simulink model "Testing_Playground"  (R2022a)
settings: Solver=VariableStepAuto  StartTime=0.0  StopTime=10.0  RelTol=1e-3
libraries: simulink x1
settings Model: Creator=maxju  LastModifiedBy=maxju

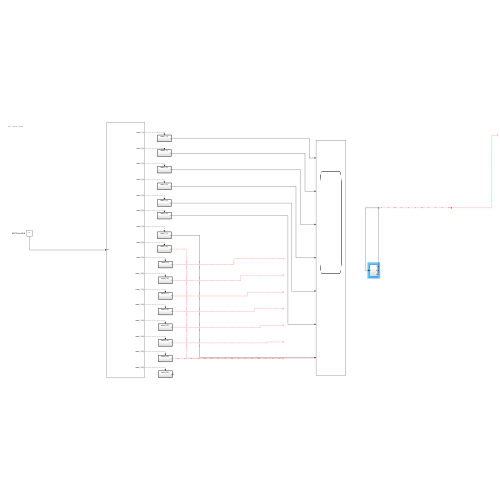
[thumbnail: Simulink's stored preview of the top-level diagram]
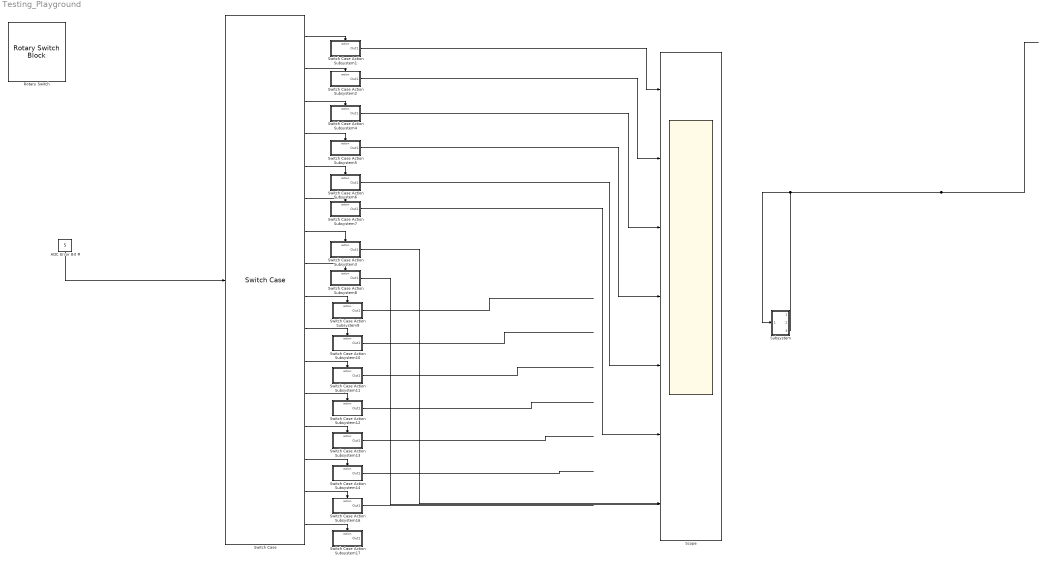
== system Testing_Playground ==
  ADC Error Bit # : Constant  Priority=0  Value=5
  Rotary Switch : RotarySwitchBlock
      settings: Values={{'No Errors', '1', '2', '3', '4', '5', '6', '7', '8', '9', '10', '11', '12', '13', '14', '15', '16'}, [0 1 2 3 4 5 6 7 8 9 10 11 12 13 14 15 16]}
  Scope : Scope  NumInputPorts=7
  Subsystem : Subsystem
  Switch Case : SwitchCase  CaseConditions={1,2,3,4,5,6,7,8,9,10,11,12,13,14,15,16}  ShowDefaultCase=off
  Switch Case Action Subsystem1 : Subsystem  TreatAsAtomicUnit=on
  Switch Case Action Subsystem10 : Subsystem  TreatAsAtomicUnit=on
  Switch Case Action Subsystem11 : Subsystem  TreatAsAtomicUnit=on
  Switch Case Action Subsystem12 : Subsystem  TreatAsAtomicUnit=on
  Switch Case Action Subsystem13 : Subsystem  TreatAsAtomicUnit=on
  Switch Case Action Subsystem14 : Subsystem  TreatAsAtomicUnit=on
  Switch Case Action Subsystem16 : Subsystem  TreatAsAtomicUnit=on
  Switch Case Action Subsystem17 : Subsystem  TreatAsAtomicUnit=on
  Switch Case Action Subsystem2 : Subsystem  TreatAsAtomicUnit=on
  Switch Case Action Subsystem3 : Subsystem  TreatAsAtomicUnit=on
  Switch Case Action Subsystem4 : Subsystem  TreatAsAtomicUnit=on
  Switch Case Action Subsystem5 : Subsystem  TreatAsAtomicUnit=on
  Switch Case Action Subsystem6 : Subsystem  TreatAsAtomicUnit=on
  Switch Case Action Subsystem7 : Subsystem  TreatAsAtomicUnit=on
  Switch Case Action Subsystem8 : Subsystem  TreatAsAtomicUnit=on
  Switch Case Action Subsystem9 : Subsystem  TreatAsAtomicUnit=on
  wires:
  Subsystem/3(Out3) -> Subsystem/1(In1)
  Switch Case Action Subsystem2/1(Out1) -> Scope/2
  Switch Case/10 -> Switch Case Action Subsystem10/Action
  Switch Case/13 -> Switch Case Action Subsystem13/Action
  Switch Case Action Subsystem16/1(Out1) -> ?
  Switch Case Action Subsystem13/1(Out1) -> ?
  Switch Case Action Subsystem9/1(Out1) -> ?
  Switch Case Action Subsystem7/1(Out1) -> Scope/6
  Switch Case/4 -> Switch Case Action Subsystem5/Action
  Switch Case Action Subsystem14/1(Out1) -> ?
  Switch Case/7 -> Switch Case Action Subsystem3/Action
  Switch Case/6 -> Switch Case Action Subsystem7/Action
  Switch Case Action Subsystem6/1(Out1) -> Scope/5
  Switch Case/3 -> Switch Case Action Subsystem4/Action
  Switch Case/15 -> Switch Case Action Subsystem16/Action
  Switch Case/14 -> Switch Case Action Subsystem14/Action
  Switch Case/12 -> Switch Case Action Subsystem12/Action
  Switch Case/5 -> Switch Case Action Subsystem6/Action
  ADC Error Bit #/1 -> Switch Case/1
  Switch Case/9 -> Switch Case Action Subsystem9/Action
  Switch Case/16 -> Switch Case Action Subsystem17/Action
  Switch Case Action Subsystem11/1(Out1) -> ?
  Switch Case Action Subsystem10/1(Out1) -> ?
  Switch Case/11 -> Switch Case Action Subsystem11/Action
  Switch Case Action Subsystem1/1(Out1) -> Scope/1
  Switch Case/2 -> Switch Case Action Subsystem2/Action
  Switch Case Action Subsystem12/1(Out1) -> ?
  Switch Case Action Subsystem4/1(Out1) -> Scope/3
  Switch Case Action Subsystem5/1(Out1) -> Scope/4
  Switch Case/8 -> Switch Case Action Subsystem8/Action
  Switch Case Action Subsystem3/1(Out1) -> Scope/7
  Switch Case Action Subsystem8/1(Out1) -> ?
  Switch Case/1 -> Switch Case Action Subsystem1/Action

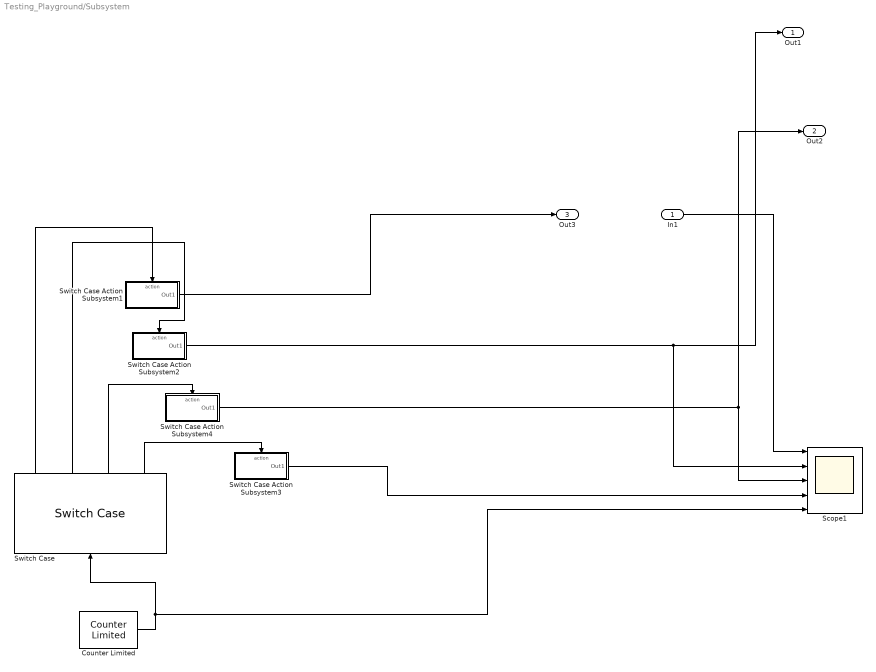
== system Testing_Playground/Subsystem ==
  In1 : Inport
  Counter Limited : simulink/Sources/Counter Limited  uplimit=3  tsamp=1
  Scope1 : Scope  NumInputPorts=5
  Switch Case : SwitchCase  CaseConditions={1,2,3}
  Switch Case Action Subsystem1 : Subsystem  TreatAsAtomicUnit=on
  Switch Case Action Subsystem2 : Subsystem  TreatAsAtomicUnit=on
  Switch Case Action Subsystem3 : Subsystem  TreatAsAtomicUnit=on
  Switch Case Action Subsystem4 : Subsystem  TreatAsAtomicUnit=on
  Out1 : Outport
  Out2 : Outport  Port=2
  Out3 : Outport  Port=3
  wires:
  Switch Case Action Subsystem4/1(Out1) -> Out2/1, Scope1/3
  Switch Case/4 -> Switch Case Action Subsystem3/Action
  Switch Case/2 -> Switch Case Action Subsystem2/Action
  Switch Case/3 -> Switch Case Action Subsystem4/Action
  Switch Case Action Subsystem3/1(Out1) -> Scope1/4
  In1/1 -> Scope1/1
  Switch Case Action Subsystem2/1(Out1) -> Out1/1, Scope1/2
  Switch Case/1 -> Switch Case Action Subsystem1/Action
  Counter Limited/1 -> Scope1/5, Switch Case/1
  Switch Case Action Subsystem1/1(Out1) -> Out3/1

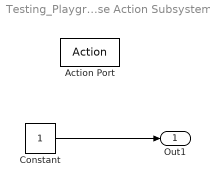
== system Testing_Playground/Switch Case Action Subsystem1 ==
  Action Port : ActionPort  ActionPortLabel=case [ 1 ]:
  Constant : Constant
  Out1 : Outport  VectorParamsAs1DForOutWhenUnconnected=off
  wires:
  Constant/1 -> Out1/1

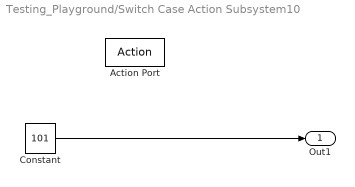
== system Testing_Playground/Switch Case Action Subsystem10 ==
  Action Port : ActionPort  ActionPortLabel=case [ 10 ]:
  Constant : Constant  Value=101
  Out1 : Outport  VectorParamsAs1DForOutWhenUnconnected=off
  wires:
  Constant/1 -> Out1/1

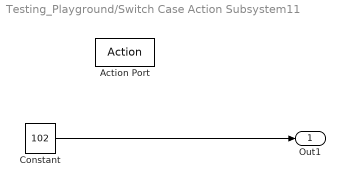
== system Testing_Playground/Switch Case Action Subsystem11 ==
  Action Port : ActionPort  ActionPortLabel=case [ 11 ]:
  Constant : Constant  Value=102
  Out1 : Outport  VectorParamsAs1DForOutWhenUnconnected=off
  wires:
  Constant/1 -> Out1/1

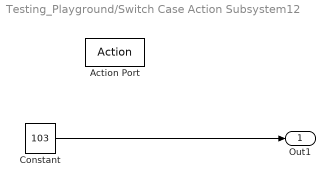
== system Testing_Playground/Switch Case Action Subsystem12 ==
  Action Port : ActionPort  ActionPortLabel=case [ 12 ]:
  Constant : Constant  Value=103
  Out1 : Outport  VectorParamsAs1DForOutWhenUnconnected=off
  wires:
  Constant/1 -> Out1/1

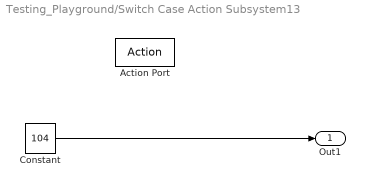
== system Testing_Playground/Switch Case Action Subsystem13 ==
  Action Port : ActionPort  ActionPortLabel=case [ 13 ]:
  Constant : Constant  Value=104
  Out1 : Outport  VectorParamsAs1DForOutWhenUnconnected=off
  wires:
  Constant/1 -> Out1/1

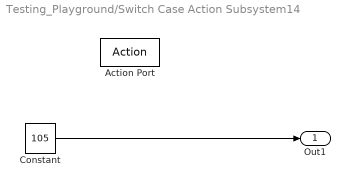
== system Testing_Playground/Switch Case Action Subsystem14 ==
  Action Port : ActionPort  ActionPortLabel=case [ 14 ]:
  Constant : Constant  Value=105
  Out1 : Outport  VectorParamsAs1DForOutWhenUnconnected=off
  wires:
  Constant/1 -> Out1/1

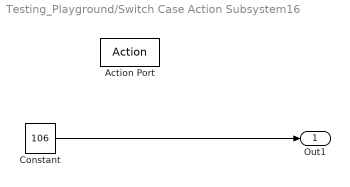
== system Testing_Playground/Switch Case Action Subsystem16 ==
  Action Port : ActionPort  ActionPortLabel=case [ 15 ]:
  Constant : Constant  Value=106
  Out1 : Outport  VectorParamsAs1DForOutWhenUnconnected=off
  wires:
  Constant/1 -> Out1/1

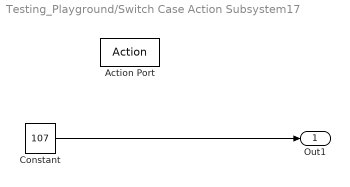
== system Testing_Playground/Switch Case Action Subsystem17 ==
  Action Port : ActionPort  ActionPortLabel=case [ 16 ]:
  Constant : Constant  Value=107
  Out1 : Outport  VectorParamsAs1DForOutWhenUnconnected=off
  wires:
  Constant/1 -> Out1/1

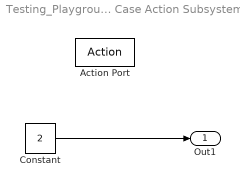
== system Testing_Playground/Switch Case Action Subsystem2 ==
  Action Port : ActionPort  ActionPortLabel=case [ 2 ]:
  Constant : Constant  Value=2
  Out1 : Outport  VectorParamsAs1DForOutWhenUnconnected=off
  wires:
  Constant/1 -> Out1/1

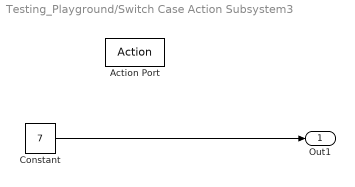
== system Testing_Playground/Switch Case Action Subsystem3 ==
  Action Port : ActionPort  ActionPortLabel=case [ 7 ]:
  Constant : Constant  Value=7
  Out1 : Outport  VectorParamsAs1DForOutWhenUnconnected=off
  wires:
  Constant/1 -> Out1/1

== system Testing_Playground/Switch Case Action Subsystem4 ==
  Action Port : ActionPort  ActionPortLabel=case [ 3 ]:
  Constant : Constant  Value=3
  Out1 : Outport  VectorParamsAs1DForOutWhenUnconnected=off
  wires:
  Constant/1 -> Out1/1

== system Testing_Playground/Switch Case Action Subsystem5 ==
  Action Port : ActionPort  ActionPortLabel=case [ 4 ]:
  Constant : Constant  Value=4
  Out1 : Outport  VectorParamsAs1DForOutWhenUnconnected=off
  wires:
  Constant/1 -> Out1/1

== system Testing_Playground/Switch Case Action Subsystem6 ==
  Action Port : ActionPort  ActionPortLabel=case [ 5 ]:
  Constant : Constant  Value=5
  Out1 : Outport  VectorParamsAs1DForOutWhenUnconnected=off
  wires:
  Constant/1 -> Out1/1

== system Testing_Playground/Switch Case Action Subsystem7 ==
  Action Port : ActionPort  ActionPortLabel=case [ 6 ]:
  Constant : Constant  Value=6
  Out1 : Outport  VectorParamsAs1DForOutWhenUnconnected=off
  wires:
  Constant/1 -> Out1/1

== system Testing_Playground/Switch Case Action Subsystem8 ==
  Action Port : ActionPort  ActionPortLabel=case [ 8 ]:
  Constant : Constant  Value=8
  Out1 : Outport  VectorParamsAs1DForOutWhenUnconnected=off
  wires:
  Constant/1 -> Out1/1

== system Testing_Playground/Switch Case Action Subsystem9 ==
  Action Port : ActionPort  ActionPortLabel=case [ 9 ]:
  Constant : Constant  Value=100
  Out1 : Outport  VectorParamsAs1DForOutWhenUnconnected=off
  wires:
  Constant/1 -> Out1/1

== system Testing_Playground/Subsystem/Switch Case Action Subsystem1 ==
  Action Port : ActionPort  InitializeStates=reset  ActionPortLabel=case [ 1 ]:
  Constant : Constant
  Out1 : Outport  VectorParamsAs1DForOutWhenUnconnected=off
  wires:
  Constant/1 -> Out1/1

== system Testing_Playground/Subsystem/Switch Case Action Subsystem2 ==
  Action Port : ActionPort  InitializeStates=reset  ActionPortLabel=case [ 2 ]:
  Constant : Constant
  Out1 : Outport  VectorParamsAs1DForOutWhenUnconnected=off
  wires:
  Constant/1 -> Out1/1

== system Testing_Playground/Subsystem/Switch Case Action Subsystem3 ==
  Action Port : ActionPort  InitializeStates=reset  ActionPortLabel=default:
  Constant : Constant  Value=0
  Out1 : Outport  VectorParamsAs1DForOutWhenUnconnected=off
  wires:
  Constant/1 -> Out1/1

== system Testing_Playground/Subsystem/Switch Case Action Subsystem4 ==
  Action Port : ActionPort  InitializeStates=reset  ActionPortLabel=case [ 3 ]:
  Constant : Constant
  Out1 : Outport  VectorParamsAs1DForOutWhenUnconnected=off
  wires:
  Constant/1 -> Out1/1
